simulink model "Top6DOFModel"  (R2018b)
settings: Solver=FixedStepAuto  StartTime=0.0  StopTime=70  FixedStep=0.005  RelTol=1e-3  EnableMultiTasking=on
InitFcn:
  | loadThrusterData
  | loadSensorData
values from neighbouring files (symbols this model uses):
  cameraVec = [1 0 0]    [loadSensorData.m]
  controlRate = 0.025    [loadBusData.m]
  controlType = 1    [loadBusData.m]    (also in loadControlData.m = 2)
  dynamicsRate = 0.005    [loadBusData.m]
  Kd = [x(4) x(5) 0 0 0 x(6)]    [executeSim.m]    (also in loadBusData.m = [500.0000  501.0938 0 0 0 18.4778]; loadControlData.m = [80 80 0 0 0 5] .*[.2 .2  0 0 0 .1]; planarPIDControl.m = [kd(1) 0 0; 0 kd(2) 0; 0 0 kd(3)])
  Ki = [x(7) x(8) 0 0 0 x(9)]    [executeSim.m]    (also in loadBusData.m = [1.0000    1.0313   0 0 0 58.1181]; loadControlData.m = [4  4  0 0 0 1] .*[1   1  0 0 0 .5]; planarPIDControl.m = [ki(1) 0 0; 0 ki(2) 0; 0 0 ki(3)])
  Kp = [x(1) x(2) 0 0 0 x(3)]    [executeSim.m]    (also in loadBusData.m = [500.0000  246.1321 0 0 0 50.1701]; loadControlData.m = [70 70 0 0 0 20].*[.2 .2  0 0 0 .25]; planarPIDControl.m = [kp(1) 0 0; 0 kp(2) 0; 0 0 kp(3)])
  rangeSensorAngBody = [0; 90*dtr; 180*dtr; 270*dtr]    [loadSensorData.m]
  rangeSensorFOV = [0*dtr; 0*dtr; 0*dtr; 0*dtr]    [loadSensorData.m]
  SMGains = x    [executeSim.m]    (also in loadBusData.m = [2.0801    3.0489    8.9333    4.9881    3.0029    9.5293   ; loadControlData.m = [3.5078    3.9888    6.3119    1.8214    4.7749    7.3059   )
  wallBounds = [wallA; wallB; wallC; wallD]    [loadSensorData.m]
undefined symbols (not defined in the file or in its folder): rangeSensorLocBody, targetVec
libraries: simulink x12
settings Model: Creator=Andy  LastModifiedBy=barthal
settings SolverCC: PositivePriorityOrder=on
settings DataIOCC: Decimation=5  SaveFormat=StructureWithTime
settings OptimizationCC: EnhancedBackFolding=on  PassReuseOutputArgsAs=Individual arguments  MaxStackSize=64  OptimizeBlockOrder=speed  DifferentSizesBufferReuse=on  OptimizationCustomize=off
settings DebuggingCC: ParameterTunabilityLossMsg=error
settings HardwareCC: ProdBitPerPointer=32  ProdBitPerSizeT=32  ProdBitPerPtrDiffT=32  ProdLargestAtomicInteger=Long  ProdLargestAtomicFloat=Double  ProdWordSize=32  ProdHWDeviceType=ARM Compatible->ARM Cortex
settings ModelReferenceCC: ModelReferenceNumInstancesAllowed=Single
settings RTWCC: SystemTargetFile=ert.tlc  HardwareBoard=Raspberry Pi  TLCOptions="-aInlineSetEventsForThisBaseRateFcn=TLC_FALSE -aSuppressMultiTaskScheduler=TLC_FALSE  -aRateBasedStepFcn=0"  GenCodeOnly=on  TemplateMakefile=ert_default_tmf  GenerateReport=on  Toolchain=GNU GCC Raspberry Pi  BuildConfiguration=Faster Runs  IncludeHyperlinkInReport=on  LaunchReport=on  TargetLang=C++  GenerateTraceInfo=on  GenerateTraceReport=on  GenerateTraceReportSl=on  GenerateTraceReportSf=on  GenerateTraceReportEml=on
settings CodeAppCC: ForceParamTrailComments=on  IgnoreCustomStorageClasses=off  OperatorAnnotations=on  SimulinkDataObjDesc=on  SFDataObjDesc=on  InsertBlockDesc=on
settings ERTTargetCC: TargetLangStandard=C++03 (ISO)  MatFileLogging=on  MultiInstanceERTCode=on  CodeInterfacePackaging=C++ class  SupportVariableSizeSignals=on  MultiInstanceErrorCode=Warning  RootIOFormat=Structure reference

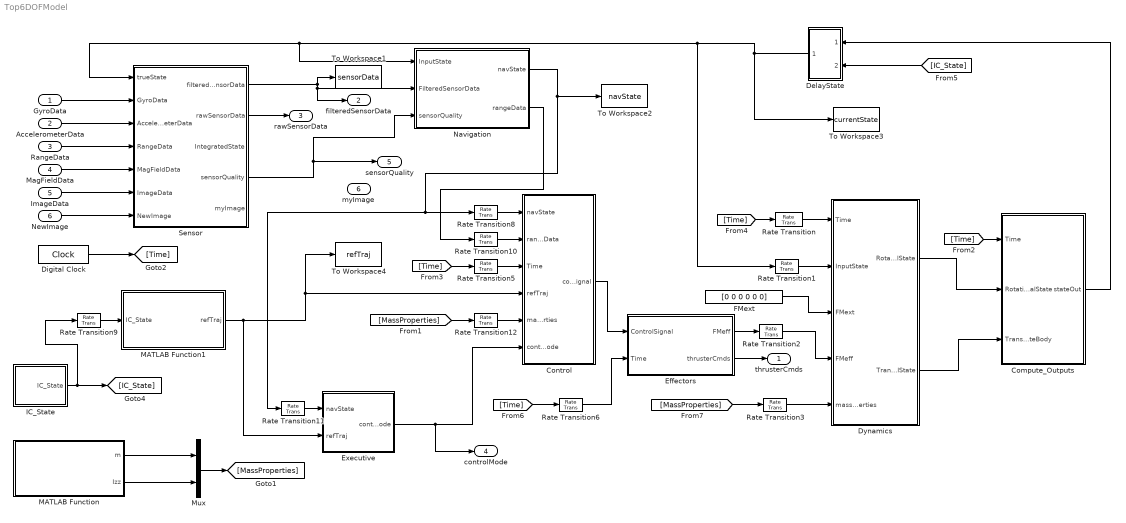
== system Top6DOFModel ==
  GyroData : Inport
  AccelerometerData : Inport  Port=2
  RangeData : Inport  Port=3  OutDataTypeStr=uint8
  MagFieldData : Inport  Port=4
  ImageData : Inport  Port=5  OutDataTypeStr=uint8  PortDimensions=[307200]
  NewImage : Inport  Port=6  OutDataTypeStr=uint8  PortDimensions=[1]
  Compute_Outputs : Subsystem
  Control : Subsystem
  DelayState : Subsystem
  Digital Clock : DigitalClock  SampleTime=0.005
  Dynamics : Subsystem  TreatAsAtomicUnit=on  SystemSampleTime=dynamicsRate
      settings: MinAlgLoopOccurrences=on
  Effectors : Subsystem  TreatAsAtomicUnit=on
  Executive : Subsystem  TreatAsAtomicUnit=on  SystemSampleTime=controlRate
  FMext : Constant  Value=[0 0 0 0 0 0]
  IC_State : Subsystem
  MATLAB Function : MATLAB Function  TreatAsAtomicUnit=on
  MATLAB Function1 : MATLAB Function  TreatAsAtomicUnit=on  SystemSampleTime=controlRate
  Mux : Mux  Inputs=2
  Navigation : Subsystem
  Rate Transition{,1..3} (4 alike) : RateTransition  OutPortSampleTime=dynamicsRate
  Rate Transition{5..6,8..12} (7 alike) : RateTransition  OutPortSampleTime=controlRate
  Sensor : Subsystem
  To Workspace1 : ToWorkspace  VariableName=sensorData  SaveFormat=Timeseries  SampleTime=-1
  To Workspace2 : ToWorkspace  VariableName=navState  SaveFormat=Timeseries  SampleTime=-1
  To Workspace3 : ToWorkspace  VariableName=currentState  SaveFormat=Timeseries  SampleTime=-1
  To Workspace4 : ToWorkspace  VariableName=refTraj  SaveFormat=Timeseries  SampleTime=-1
  thrusterCmds : Outport
  filteredSensorData : Outport  Port=2  OutDataTypeStr=double
  rawSensorData : Outport  Port=3  OutDataTypeStr=double
  controlMode : Outport  Port=4
  sensorQuality : Outport  Port=5
  myImage : Outport  Port=6
  wires:
  Digital Clock/1 -> [Time]
  FMext/1 -> Dynamics/3(FMext)
  Control/1(controlSignal) -> Effectors/1(ControlSignal)
  Dynamics/1(RotationalState) -> Compute_Outputs/2(RotationalState)
  Rate Transition/1 -> Dynamics/1(Time)
  Rate Transition1/1 -> Dynamics/2(InputState)
  Effectors/1(FMeff) -> Rate Transition2/1
  Rate Transition2/1 -> Dynamics/4(FMeff)
  Rate Transition3/1 -> Dynamics/5(massProperties)
  Rate Transition5/1 -> Control/3(Time)
  Rate Transition6/1 -> Effectors/2(Time)
  Dynamics/2(TranslationalState) -> Compute_Outputs/3(TranslationalStateBody)
  IC_State/1(IC_State) -> [IC_State], Rate Transition9/1
  Compute_Outputs/1(stateOut) -> DelayState/1(In4)
  [IC_State] -> DelayState/2(In12)
  DelayState/1(Out4) -> Rate Transition1/1, Navigation/1(InputState), Sensor/1(trueState), To Workspace3/1
  [Time] -> Compute_Outputs/1(Time)
  Rate Transition8/1 -> Control/1(navState)
  MATLAB Function1/1(refTraj) -> To Workspace4/1, Control/4(refTraj), Executive/2(refTraj)
  Effectors/2(thrusterCmds) -> thrusterCmds/1
  GyroData/1 -> Sensor/2(GyroData)
  AccelerometerData/1 -> Sensor/3(AccelerometerData)
  RangeData/1 -> Sensor/4(RangeData)
  Sensor/1(filteredSensorData) -> filteredSensorData/1, Navigation/2(FilteredSensorData), To Workspace1/1
  Executive/1(controlMode) -> Control/6(controlMode), controlMode/1
  Rate Transition11/1 -> Executive/1(navState)
  Rate Transition9/1 -> MATLAB Function1/1(IC_State)
  Rate Transition10/1 -> Control/2(rangeData)
  [Time] -> Rate Transition5/1
  MagFieldData/1 -> Sensor/5(MagFieldData)
  Navigation/1(navState) -> To Workspace2/1, Rate Transition11/1, Rate Transition8/1
  Navigation/2(rangeData) -> Rate Transition10/1
  [Time] -> Rate Transition/1
  [Time] -> Rate Transition6/1
  Sensor/2(rawSensorData) -> rawSensorData/1
  Rate Transition12/1 -> Control/5(massProperties)
  Mux/1 -> [MassProperties]
  [MassProperties] -> Rate Transition12/1
  [MassProperties] -> Rate Transition3/1
  MATLAB Function/1(m) -> Mux/1
  MATLAB Function/2(Izz) -> Mux/2
  Sensor/4(sensorQuality) -> sensorQuality/1, Navigation/3(sensorQuality)
  ImageData/1 -> Sensor/6(ImageData)
  NewImage/1 -> Sensor/7(NewImage)

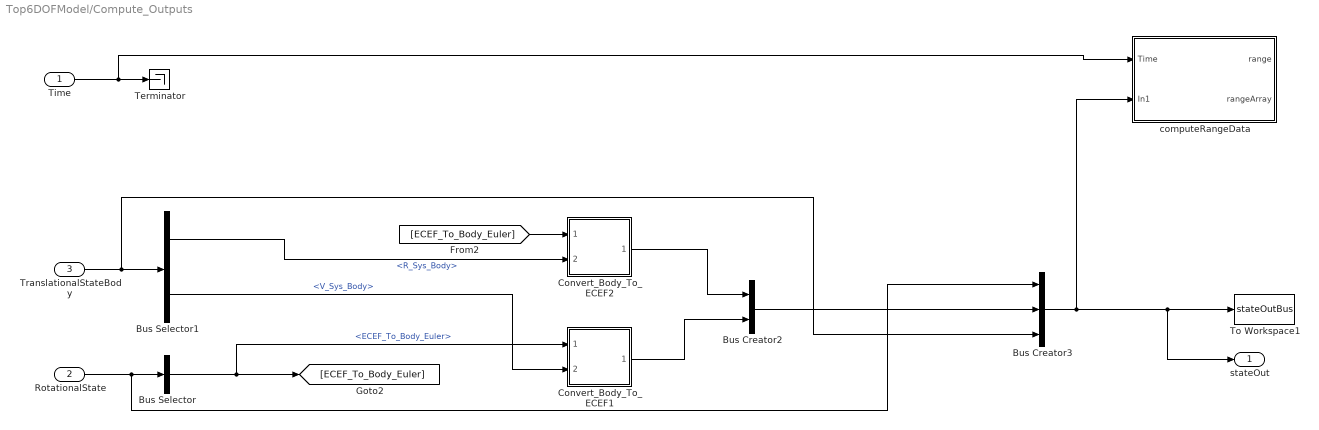
== system Top6DOFModel/Compute_Outputs ==
  Time : Inport
  RotationalState : Inport  Port=2
  TranslationalStateBody : Inport  Port=3
  Bus Creator2 : BusCreator  Inputs=2  OutDataTypeStr=Bus: TranStateECEFBus
      settings: InheritFromInputs=off
  Bus Creator3 : BusCreator  Inputs=3  OutDataTypeStr=Bus: FullStateBus
      settings: InheritFromInputs=off
  Bus Selector : BusSelector  OutputSignals=ECEF_To_Body_Euler
  Bus Selector1 : BusSelector  OutputSignals=R_Sys_Body,V_Sys_Body
  Convert_Body_To_ECEF1 : Subsystem
  Convert_Body_To_ECEF2 : Subsystem
  Terminator : Terminator
  To Workspace1 : ToWorkspace  VariableName=stateOutBus  SaveFormat=Timeseries  SampleTime=-1
  computeRangeData : Subsystem
  stateOut : Outport
  wires:
  RotationalState/1 -> Bus Creator3/1, Bus Selector/1
  Bus Selector/1 -> Convert_Body_To_ECEF1/1(ECEF_To_Body_Euler), [ECEF_To_Body_Euler]  "<ECEF_To_Body_Euler>"
  Convert_Body_To_ECEF2/1(Vec_ECEF) -> Bus Creator2/1
  Convert_Body_To_ECEF1/1(Vec_ECEF) -> Bus Creator2/2
  [ECEF_To_Body_Euler] -> Convert_Body_To_ECEF2/1(ECEF_To_Body_Euler)
  TranslationalStateBody/1 -> Bus Creator3/3, Bus Selector1/1
  Bus Selector1/1 -> Convert_Body_To_ECEF2/2(Vec_Body)  "<R_Sys_Body>"
  Bus Selector1/2 -> Convert_Body_To_ECEF1/2(Vec_Body)  "<V_Sys_Body>"
  Bus Creator2/1 -> Bus Creator3/2
  Bus Creator3/1 -> stateOut/1, To Workspace1/1, computeRangeData/2(In1)
  Time/1 -> computeRangeData/1(Time), Terminator/1

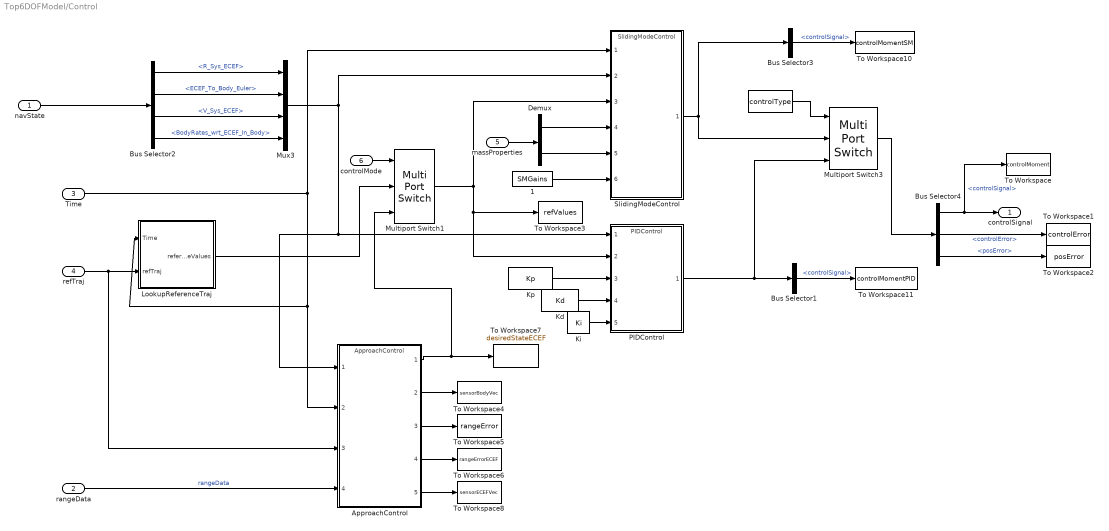
== system Top6DOFModel/Control ==
  navState : Inport
  rangeData : Inport  Port=2
  Time : Inport  Port=3
  refTraj : Inport  Port=4
  massProperties : Inport  Port=5
  controlMode : Inport  Port=6
  " " : Constant  Value=controlType
  " 1" : Constant  Value=SMGains
  ApproachControl : ModelReference  ModelNameDialog=ApproachControl  SimulationMode=Normal  ModelReferenceVersion=1.58
  Bus Selector1 : BusSelector  OutputSignals=controlSignal
  Bus Selector2 : BusSelector  OutputSignals=TranState_ECEF.R_Sys_ECEF,RotState_Body_ECEF.ECEF_To_Body_Euler,TranState_ECEF.V_Sys_ECEF,RotState_Body_ECEF.BodyRates_wrt_ECEF_In_Body
  Bus Selector3 : BusSelector  OutputSignals=controlSignal
  Bus Selector4 : BusSelector  OutputSignals=controlSignal,controlError,posError
  Demux : Demux  Outputs=2
  Kd : Constant  Value=Kd
  Ki : Constant  Value=Ki
  Kp : Constant  Value=Kp
  LookupReferenceTraj : Subsystem
  Multiport Switch1 : MultiPortSwitch  Inputs=2
  Multiport Switch3 : MultiPortSwitch  Inputs=2
  Mux3 : Mux
  PIDControl : ModelReference  ModelNameDialog=PIDControl  SimulationMode=Normal  ModelReferenceVersion=1.353
  SlidingModeControl : ModelReference  ModelNameDialog=SlidingModeControl  SimulationMode=Normal  ModelReferenceVersion=1.17
  To Workspace : ToWorkspace  VariableName=controlMoment  SaveFormat=Timeseries  SampleTime=-1
  To Workspace1 : ToWorkspace  VariableName=controlError  SaveFormat=Timeseries  SampleTime=-1
  To Workspace10 : ToWorkspace  VariableName=controlMomentSM  SaveFormat=Timeseries  SampleTime=-1
  To Workspace11 : ToWorkspace  VariableName=controlMomentPID  SaveFormat=Timeseries  SampleTime=-1
  To Workspace2 : ToWorkspace  VariableName=posError  SaveFormat=Timeseries  SampleTime=-1
  To Workspace3 : ToWorkspace  VariableName=refValues  SaveFormat=Timeseries  SampleTime=-1
  To Workspace4 : ToWorkspace  VariableName=sensorBodyVec  SaveFormat=Timeseries  SampleTime=-1
  To Workspace5 : ToWorkspace  VariableName=rangeError  SaveFormat=Timeseries  SampleTime=-1
  To Workspace6 : ToWorkspace  VariableName=rangeErrorECEF  SaveFormat=Timeseries  SampleTime=-1
  To Workspace7 : ToWorkspace  VariableName=desiredStateECEF  SaveFormat=Timeseries  SampleTime=-1
  To Workspace8 : ToWorkspace  VariableName=sensorECEFVec  SaveFormat=Timeseries  SampleTime=-1
  controlSignal : Outport
  wires:
  refTraj/1 -> LookupReferenceTraj/2(refTraj), ApproachControl/3
  Mux3/1 -> SlidingModeControl/2, PIDControl/1, ApproachControl/1
  navState/1 -> Bus Selector2/1
  Bus Selector2/1 -> Mux3/1  "<R_Sys_ECEF>"
  Bus Selector2/2 -> Mux3/2  "<ECEF_To_Body_Euler>"
  Bus Selector2/3 -> Mux3/3  "<V_Sys_ECEF>"
  Bus Selector2/4 -> Mux3/4  "<BodyRates_wrt_ECEF_In_Body>"
  rangeData/1 -> ApproachControl/4  "rangeData"
  Time/1 -> ApproachControl/2, LookupReferenceTraj/1(Time), SlidingModeControl/1
  Kp/1 -> PIDControl/3
  Kd/1 -> PIDControl/4
  Ki/1 -> PIDControl/5
  Demux/2 -> SlidingModeControl/5
  SlidingModeControl/1 -> Bus Selector3/1, Multiport Switch3/2
  " "/1 -> Multiport Switch3/1
  PIDControl/1 -> Bus Selector1/1, Multiport Switch3/3
  Multiport Switch3/1 -> Bus Selector4/1
  Bus Selector4/1 -> To Workspace/1, controlSignal/1  "<controlSignal>"
  Bus Selector4/2 -> To Workspace1/1  "<controlError>"
  Bus Selector4/3 -> To Workspace2/1  "<posError>"
  Bus Selector1/1 -> To Workspace11/1  "<controlSignal>"
  Bus Selector3/1 -> To Workspace10/1  "<controlSignal>"
  " 1"/1 -> SlidingModeControl/6
  controlMode/1 -> Multiport Switch1/1
  Multiport Switch1/1 -> To Workspace3/1, PIDControl/2, SlidingModeControl/3
  LookupReferenceTraj/1(referenceValues) -> Multiport Switch1/2
  ApproachControl/1 -> Multiport Switch1/3, To Workspace7/1
  ApproachControl/2 -> To Workspace4/1
  ApproachControl/3 -> To Workspace5/1
  ApproachControl/4 -> To Workspace6/1
  ApproachControl/5 -> To Workspace8/1
  Demux/1 -> SlidingModeControl/4
  massProperties/1 -> Demux/1

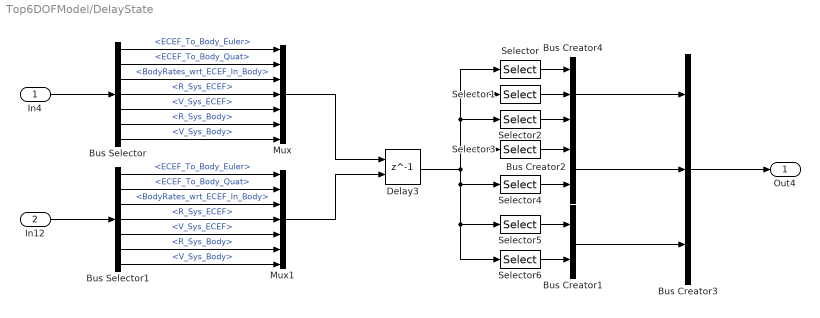
== system Top6DOFModel/DelayState ==
  In4 : Inport
  In12 : Inport  Port=2
  Bus Creator1 : BusCreator  Inputs=2  OutDataTypeStr=Bus: TranStateBodyBus
      settings: InheritFromInputs=off
  Bus Creator2 : BusCreator  Inputs=2  OutDataTypeStr=Bus: TranStateECEFBus
      settings: InheritFromInputs=off
  Bus Creator3 : BusCreator  Inputs=3  OutDataTypeStr=Bus: FullStateBus
      settings: InheritFromInputs=off
  Bus Creator4 : BusCreator  Inputs=3  OutDataTypeStr=Bus: RotStateBodyECEFBus
      settings: InheritFromInputs=off
  Bus Selector : BusSelector  OutputSignals=RotState_Body_ECEF.ECEF_To_Body_Euler,RotState_Body_ECEF.ECEF_To_Body_Quat,RotState_Body_ECEF.BodyRates_wrt_ECEF_In_Body,TranState_ECEF.R_Sys_ECEF,TranState_ECEF.V_Sys_ECEF,TranState_Body.R_Sys_Body,TranState_Body.V_Sys_Body
  Bus Selector1 : BusSelector  OutputSignals=RotState_Body_ECEF.ECEF_To_Body_Euler,RotState_Body_ECEF.ECEF_To_Body_Quat,RotState_Body_ECEF.BodyRates_wrt_ECEF_In_Body,TranState_ECEF.R_Sys_ECEF,TranState_ECEF.V_Sys_ECEF,TranState_Body.R_Sys_Body,TranState_Body.V_Sys_Body
  Delay3 : Delay  DelayLength=1  InitialConditionSource=Input port
      settings: InputPortMap=u0,p4
  Mux : Mux  Inputs=7
  Mux1 : Mux  Inputs=7
  Selector : Selector  InputPortWidth=22  IndexOptions=Index vector (dialog)  Indices=[1:3]  OutputSizes=1
  Selector1 : Selector  InputPortWidth=22  IndexOptions=Index vector (dialog)  Indices=[4:7]  OutputSizes=1
  Selector2 : Selector  InputPortWidth=22  IndexOptions=Index vector (dialog)  Indices=[8:10]  OutputSizes=1
  Selector3 : Selector  InputPortWidth=22  IndexOptions=Index vector (dialog)  Indices=[11:13]  OutputSizes=1
  Selector4 : Selector  InputPortWidth=22  IndexOptions=Index vector (dialog)  Indices=[14:16]  OutputSizes=1
  Selector5 : Selector  InputPortWidth=22  IndexOptions=Index vector (dialog)  Indices=[17:19]  OutputSizes=1
  Selector6 : Selector  InputPortWidth=22  IndexOptions=Index vector (dialog)  Indices=[20:22]  OutputSizes=1
  Out4 : Outport
  wires:
  Bus Creator3/1 -> Out4/1
  Bus Creator1/1 -> Bus Creator3/3
  Bus Creator2/1 -> Bus Creator3/2
  Bus Creator4/1 -> Bus Creator3/1
  In4/1 -> Bus Selector/1
  Bus Selector/1 -> Mux/1  "<ECEF_To_Body_Euler>"
  Bus Selector/2 -> Mux/2  "<ECEF_To_Body_Quat>"
  Bus Selector/3 -> Mux/3  "<BodyRates_wrt_ECEF_In_Body>"
  Bus Selector/4 -> Mux/4  "<R_Sys_ECEF>"
  Bus Selector/5 -> Mux/5  "<V_Sys_ECEF>"
  Bus Selector/6 -> Mux/6  "<R_Sys_Body>"
  Bus Selector/7 -> Mux/7  "<V_Sys_Body>"
  Bus Selector1/4 -> Mux1/4  "<R_Sys_ECEF>"
  Bus Selector1/2 -> Mux1/2  "<ECEF_To_Body_Quat>"
  Bus Selector1/1 -> Mux1/1  "<ECEF_To_Body_Euler>"
  In12/1 -> Bus Selector1/1
  Bus Selector1/6 -> Mux1/6  "<R_Sys_Body>"
  Bus Selector1/5 -> Mux1/5  "<V_Sys_ECEF>"
  Bus Selector1/7 -> Mux1/7  "<V_Sys_Body>"
  Bus Selector1/3 -> Mux1/3  "<BodyRates_wrt_ECEF_In_Body>"
  Mux/1 -> Delay3/1
  Mux1/1 -> Delay3/2
  Selector/1 -> Bus Creator4/1
  Selector1/1 -> Bus Creator4/2
  Selector2/1 -> Bus Creator4/3
  Selector3/1 -> Bus Creator2/1
  Selector4/1 -> Bus Creator2/2
  Selector5/1 -> Bus Creator1/1
  Selector6/1 -> Bus Creator1/2
  Delay3/1 -> Selector/1, Selector1/1, Selector2/1, Selector3/1, Selector4/1, Selector5/1, Selector6/1

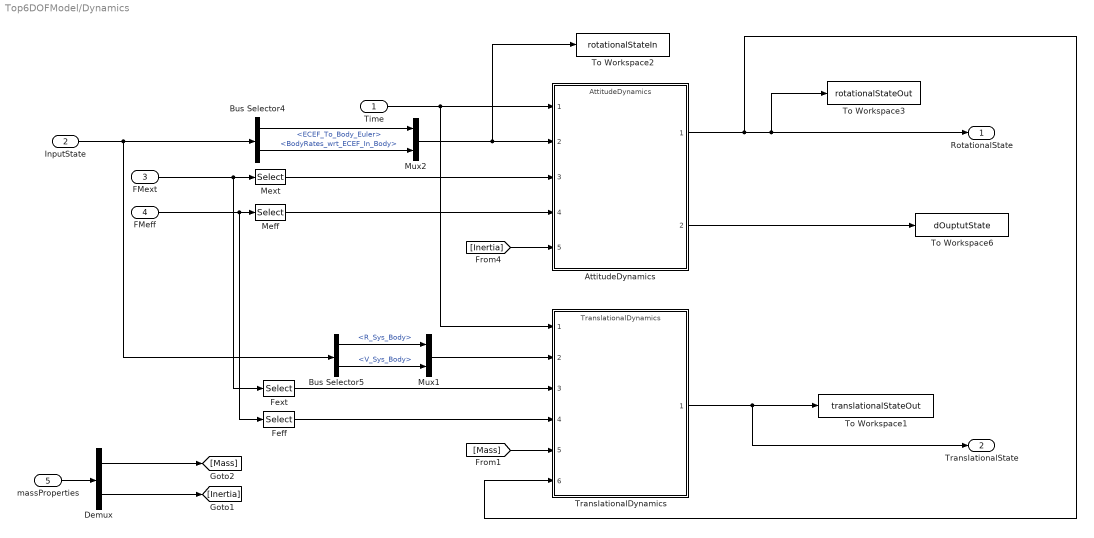
== system Top6DOFModel/Dynamics ==
  Time : Inport
  InputState : Inport  Port=2
  FMext : Inport  Port=3
  FMeff : Inport  Port=4
  massProperties : Inport  Port=5
  AttitudeDynamics : ModelReference  ModelNameDialog=AttitudeDynamics  SimulationMode=Normal  ModelReferenceVersion=1.377
  Bus Selector4 : BusSelector  OutputSignals=RotState_Body_ECEF.ECEF_To_Body_Euler,RotState_Body_ECEF.BodyRates_wrt_ECEF_In_Body
  Bus Selector5 : BusSelector  OutputSignals=TranState_Body.R_Sys_Body,TranState_Body.V_Sys_Body
  Demux : Demux  Outputs=2
  Feff : Selector  InputPortWidth=6  IndexOptions=Index vector (dialog)  Indices=[1:3]  OutputSizes=1
  Fext : Selector  InputPortWidth=6  IndexOptions=Index vector (dialog)  Indices=[1:3]  OutputSizes=1
  Meff : Selector  InputPortWidth=6  IndexOptions=Index vector (dialog)  Indices=[4:6]  OutputSizes=1
  Mext : Selector  InputPortWidth=6  IndexOptions=Index vector (dialog)  Indices=[4:6]  OutputSizes=1
  Mux1 : Mux  Inputs=2
  Mux2 : Mux  Inputs=2
  To Workspace1 : ToWorkspace  VariableName=translationalStateOut  SaveFormat=Timeseries  SampleTime=-1
  To Workspace2 : ToWorkspace  VariableName=rotationalStateIn  SaveFormat=Timeseries  SampleTime=-1
  To Workspace3 : ToWorkspace  VariableName=rotationalStateOut  SaveFormat=Timeseries  SampleTime=-1
  To Workspace6 : ToWorkspace  VariableName=dOuptutState  SaveFormat=Timeseries  SampleTime=-1
  TranslationalDynamics : ModelReference  ModelNameDialog=TranslationalDynamics  SimulationMode=Normal  ModelReferenceVersion=1.363
  RotationalState : Outport
  TranslationalState : Outport  Port=2
  wires:
  Time/1 -> AttitudeDynamics/1, TranslationalDynamics/1
  FMext/1 -> Mext/1, Fext/1
  Mext/1 -> AttitudeDynamics/3
  Fext/1 -> TranslationalDynamics/3
  FMeff/1 -> Feff/1, Meff/1
  Feff/1 -> TranslationalDynamics/4
  Meff/1 -> AttitudeDynamics/4
  AttitudeDynamics/2 -> To Workspace6/1
  AttitudeDynamics/1 -> RotationalState/1, To Workspace3/1, TranslationalDynamics/6
  TranslationalDynamics/1 -> TranslationalState/1, To Workspace1/1
  InputState/1 -> Bus Selector5/1, Bus Selector4/1
  Bus Selector4/1 -> Mux2/1  "<ECEF_To_Body_Euler>"
  Bus Selector4/2 -> Mux2/2  "<BodyRates_wrt_ECEF_In_Body>"
  Mux1/1 -> TranslationalDynamics/2
  Mux2/1 -> To Workspace2/1, AttitudeDynamics/2
  Bus Selector5/1 -> Mux1/1  "<R_Sys_Body>"
  Bus Selector5/2 -> Mux1/2  "<V_Sys_Body>"
  massProperties/1 -> Demux/1
  [Inertia] -> AttitudeDynamics/5
  [Mass] -> TranslationalDynamics/5
  Demux/1 -> [Mass]
  Demux/2 -> [Inertia]

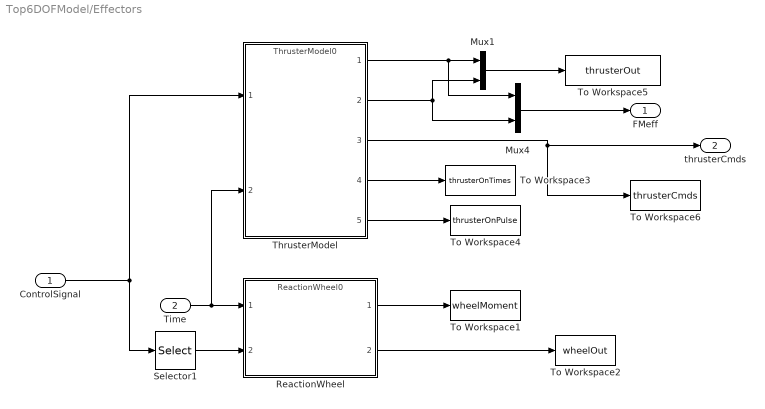
== system Top6DOFModel/Effectors ==
  ControlSignal : Inport
  Time : Inport  Port=2
  Mux1 : Mux  Inputs=2
  Mux4 : Mux  Inputs=2
  ReactionWheel : ModelReference  ModelNameDialog=ReactionWheel0  SimulationMode=Normal  ModelReferenceVersion=1.304
  Selector1 : Selector  InputPortWidth=6  IndexOptions=Index vector (dialog)  Indices=[6]  OutputSizes=1
  ThrusterModel : ModelReference  ModelNameDialog=ThrusterModel0  SimulationMode=Normal  ModelReferenceVersion=1.328
  To Workspace1 : ToWorkspace  VariableName=wheelMoment  SaveFormat=Timeseries  SampleTime=-1
  To Workspace2 : ToWorkspace  VariableName=wheelOut  SaveFormat=Timeseries  SampleTime=-1
  To Workspace3 : ToWorkspace  VariableName=thrusterOnTimes  SaveFormat=Timeseries  SampleTime=-1
  To Workspace4 : ToWorkspace  VariableName=thrusterOnPulse  SaveFormat=Timeseries  SampleTime=-1
  To Workspace5 : ToWorkspace  VariableName=thrusterOut  SaveFormat=Timeseries  SampleTime=-1
  To Workspace6 : ToWorkspace  VariableName=thrusterCmds  SaveFormat=Timeseries  SampleTime=-1
  FMeff : Outport
  thrusterCmds : Outport  Port=2
  wires:
  Selector1/1 -> ReactionWheel/2
  ControlSignal/1 -> ThrusterModel/1, Selector1/1
  Time/1 -> ThrusterModel/2, ReactionWheel/1
  Mux4/1 -> FMeff/1
  ThrusterModel/3 -> To Workspace6/1, thrusterCmds/1
  ReactionWheel/1 -> To Workspace1/1
  ReactionWheel/2 -> To Workspace2/1
  ThrusterModel/2 -> Mux4/2, Mux1/2
  ThrusterModel/1 -> Mux4/1, Mux1/1
  Mux1/1 -> To Workspace5/1
  ThrusterModel/4 -> To Workspace3/1
  ThrusterModel/5 -> To Workspace4/1

== system Top6DOFModel/Executive ==
  navState : Inport
  refTraj : Inport  Port=2
  Constant : Constant
  Delay : Delay  DelayLength=1  InitialConditionSource=Input port  InitialCondition=0
      settings: InputPortMap=u0,p4
  MATLAB Function : MATLAB Function  TreatAsAtomicUnit=on
  To Workspace2 : ToWorkspace  VariableName=controlMode  SaveFormat=Timeseries  SampleTime=-1
  controlMode : Outport
  wires:
  Delay/1 -> MATLAB Function/3(inControlMode)
  refTraj/1 -> MATLAB Function/2(refTraj)
  navState/1 -> MATLAB Function/1(navState)
  MATLAB Function/1(outControlMode) -> To Workspace2/1, controlMode/1, Delay/1
  Constant/1 -> Delay/2

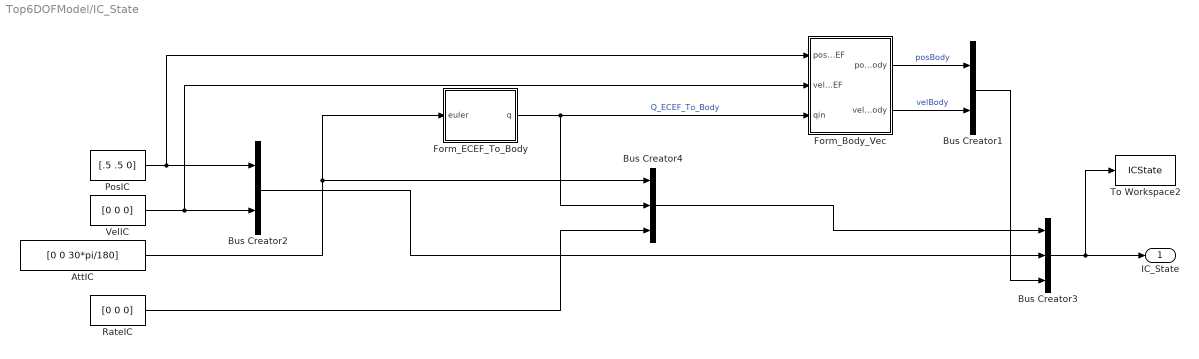
== system Top6DOFModel/IC_State ==
  AttIC : Constant  Value=[0 0 30*pi/180]
  Bus Creator1 : BusCreator  Inputs=2  OutDataTypeStr=Bus: TranStateBodyBus
      settings: InheritFromInputs=off
  Bus Creator2 : BusCreator  Inputs=2  OutDataTypeStr=Bus: TranStateECEFBus
      settings: InheritFromInputs=off
  Bus Creator3 : BusCreator  Inputs=3  OutDataTypeStr=Bus: FullStateBus
      settings: InheritFromInputs=off
  Bus Creator4 : BusCreator  Inputs=3  OutDataTypeStr=Bus: RotStateBodyECEFBus
      settings: InheritFromInputs=off
  Form_Body_Vec : MATLAB Function  TreatAsAtomicUnit=on
  Form_ECEF_To_Body : MATLAB Function  TreatAsAtomicUnit=on
  PosIC : Constant  Value=[.5 .5 0]
  RateIC : Constant  Value=[0 0 0]
  To Workspace2 : ToWorkspace  VariableName=ICState  SaveFormat=Timeseries  SampleTime=-1
  VelIC : Constant  Value=[0 0 0]
  IC_State : Outport
  wires:
  RateIC/1 -> Bus Creator4/3
  PosIC/1 -> Form_Body_Vec/1(posECEF), Bus Creator2/1
  VelIC/1 -> Bus Creator2/2, Form_Body_Vec/2(velECEF)
  Form_ECEF_To_Body/1(q) -> Form_Body_Vec/3(qin), Bus Creator4/2  "Q_ECEF_To_Body"
  Form_Body_Vec/1(posBody) -> Bus Creator1/1  "posBody"
  Form_Body_Vec/2(velBody) -> Bus Creator1/2  "velBody"
  Bus Creator2/1 -> Bus Creator3/2
  Bus Creator1/1 -> Bus Creator3/3
  Bus Creator4/1 -> Bus Creator3/1
  Bus Creator3/1 -> To Workspace2/1, IC_State/1
  AttIC/1 -> Bus Creator4/1, Form_ECEF_To_Body/1(euler)

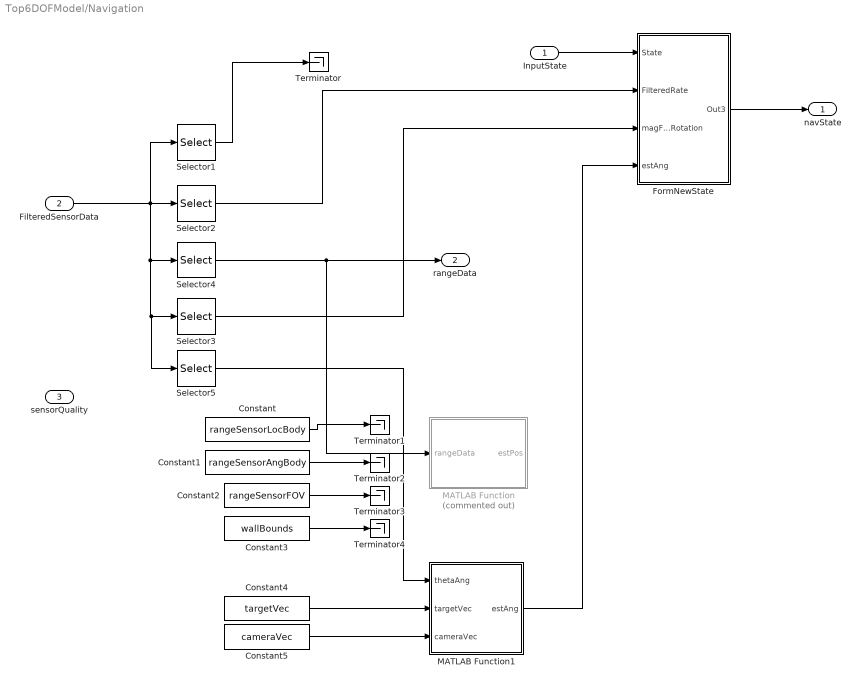
== system Top6DOFModel/Navigation ==
  InputState : Inport
  FilteredSensorData : Inport  Port=2
  sensorQuality : Inport  Port=3
  Constant : Constant  Value=rangeSensorLocBody
  Constant1 : Constant  Value=rangeSensorAngBody
  Constant2 : Constant  Value=rangeSensorFOV
  Constant3 : Constant  Value=wallBounds
  Constant4 : Constant  Value=targetVec
  Constant5 : Constant  Value=cameraVec
  FormNewState : Subsystem
  MATLAB Function : MATLAB Function  Commented=on  TreatAsAtomicUnit=on
  MATLAB Function1 : MATLAB Function  TreatAsAtomicUnit=on
  Selector1 : Selector  InputPortWidth=14  IndexOptions=Index vector (dialog)  Indices=[1:3]  OutputSizes=1
  Selector2 : Selector  InputPortWidth=14  IndexOptions=Index vector (dialog)  Indices=[4:6]  OutputSizes=1
  Selector3 : Selector  InputPortWidth=14  IndexOptions=Index vector (dialog)  Indices=[11:13]  OutputSizes=1
  Selector4 : Selector  InputPortWidth=14  IndexOptions=Index vector (dialog)  Indices=[7:10]  OutputSizes=1
  Selector5 : Selector  InputPortWidth=14  IndexOptions=Index vector (dialog)  Indices=[14]  OutputSizes=1
  Terminator{,1..4} (5 alike) : Terminator
  navState : Outport
  rangeData : Outport  Port=2
  wires:
  FilteredSensorData/1 -> Selector4/1, Selector5/1, Selector3/1, Selector2/1, Selector1/1
  Selector2/1 -> FormNewState/2(FilteredRate)
  Selector3/1 -> FormNewState/3(magFieldRotation)
  InputState/1 -> FormNewState/1(State)
  FormNewState/1(Out3) -> navState/1
  Selector4/1 -> MATLAB Function/1(rangeData), rangeData/1
  Constant3/1 -> Terminator4/1
  Constant2/1 -> Terminator3/1
  Constant1/1 -> Terminator2/1
  Constant/1 -> Terminator1/1
  Selector1/1 -> Terminator/1
  Selector5/1 -> MATLAB Function1/1(thetaAng)
  Constant4/1 -> MATLAB Function1/2(targetVec)
  MATLAB Function1/1(estAng) -> FormNewState/4(estAng)
  Constant5/1 -> MATLAB Function1/3(cameraVec)

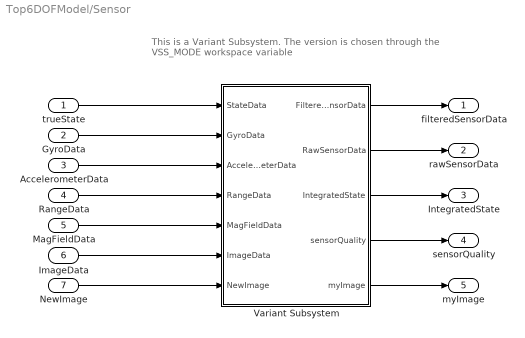
== system Top6DOFModel/Sensor ==
  note: This is a Variant Subsystem.
      | The version is chosen through the VSS_MODE workspace variable
  trueState : Inport  OutDataTypeStr=double
  GyroData : Inport  Port=2  OutDataTypeStr=double
  AccelerometerData : Inport  Port=3  OutDataTypeStr=double
  RangeData : Inport  Port=4  OutDataTypeStr=uint8
  MagFieldData : Inport  Port=5  OutDataTypeStr=double
  ImageData : Inport  Port=6
  NewImage : Inport  Port=7  OutDataTypeStr=uint8
  Variant Subsystem : Subsystem  Variant=on
  filteredSensorData : Outport  OutDataTypeStr=double
  rawSensorData : Outport  Port=2  OutDataTypeStr=double
  IntegratedState : Outport  Port=3  OutDataTypeStr=double
  sensorQuality : Outport  Port=4
  myImage : Outport  Port=5  OutDataTypeStr=uint8
  wires:
  trueState/1 -> Variant Subsystem/1(StateData)
  GyroData/1 -> Variant Subsystem/2(GyroData)
  AccelerometerData/1 -> Variant Subsystem/3(AccelerometerData)
  RangeData/1 -> Variant Subsystem/4(RangeData)
  Variant Subsystem/1(FilteredSensorData) -> filteredSensorData/1
  MagFieldData/1 -> Variant Subsystem/5(MagFieldData)
  Variant Subsystem/2(RawSensorData) -> rawSensorData/1
  Variant Subsystem/3(IntegratedState) -> IntegratedState/1
  Variant Subsystem/4(sensorQuality) -> sensorQuality/1
  ImageData/1 -> Variant Subsystem/6(ImageData)
  Variant Subsystem/5(myImage) -> myImage/1
  NewImage/1 -> Variant Subsystem/7(NewImage)

== system Top6DOFModel/Compute_Outputs/Convert_Body_To_ECEF1 ==
  ECEF_To_Body_Euler : Inport
  Vec_Body : Inport  Port=2  PortDimensions=3
  Form_ECEF_To_Body : MATLAB Function  TreatAsAtomicUnit=on
  Math Function : Math  Operator=transpose  SaturateOnIntegerOverflow=on
  Product : Product  Multiplication=Matrix(*)
  Terminator : Terminator
  Vec_ECEF : Outport  PortDimensions=3
  wires:
  Form_ECEF_To_Body/1(m) -> Math Function/1  "M_ECEF_To_Body"
  Vec_Body/1 -> Product/2
  Product/1 -> Vec_ECEF/1
  ECEF_To_Body_Euler/1 -> Form_ECEF_To_Body/1(euler)
  Form_ECEF_To_Body/2(q) -> Terminator/1  "q_ECEF_To_Body"
  Math Function/1 -> Product/1

== system Top6DOFModel/Compute_Outputs/Convert_Body_To_ECEF2 ==
  ECEF_To_Body_Euler : Inport
  Vec_Body : Inport  Port=2  PortDimensions=3
  Form_ECEF_To_Body : MATLAB Function  TreatAsAtomicUnit=on
  Math Function : Math  Operator=transpose  SaturateOnIntegerOverflow=on
  Product : Product  Multiplication=Matrix(*)
  Terminator : Terminator
  Vec_ECEF : Outport  PortDimensions=3
  wires:
  Form_ECEF_To_Body/1(m) -> Math Function/1  "M_ECEF_To_Body"
  Vec_Body/1 -> Product/2
  Product/1 -> Vec_ECEF/1
  ECEF_To_Body_Euler/1 -> Form_ECEF_To_Body/1(euler)
  Form_ECEF_To_Body/2(q) -> Terminator/1  "q_ECEF_To_Body"
  Math Function/1 -> Product/1

== system Top6DOFModel/Compute_Outputs/computeRangeData ==
  Time : Inport
  In1 : Inport  Port=2
  Constant : Constant  Value=rangeSensorLocBody
  Constant1 : Constant  Value=rangeSensorAngBody
  Constant2 : Constant  Value=rangeSensorFOV
  Constant3 : Constant  Value=wallBounds
  MATLAB Function1 : MATLAB Function  TreatAsAtomicUnit=on
  range : Outport
  rangeArray : Outport  Port=2
  wires:
  In1/1 -> MATLAB Function1/2(state)
  Constant/1 -> MATLAB Function1/3(rangeSensorLocBody)
  Constant1/1 -> MATLAB Function1/4(rangeSensorAngBody)
  Constant2/1 -> MATLAB Function1/5(rangeSensorFOV)
  MATLAB Function1/1(range) -> range/1
  Constant3/1 -> MATLAB Function1/6(wallBounds)
  MATLAB Function1/2(rangeArray) -> rangeArray/1
  Time/1 -> MATLAB Function1/1(t)

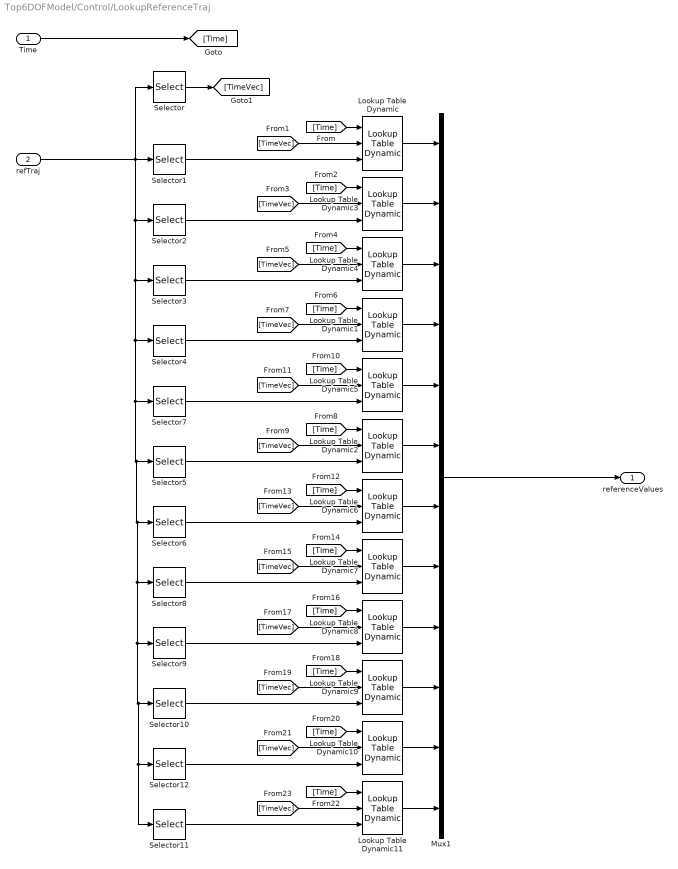
== system Top6DOFModel/Control/LookupReferenceTraj ==
  Time : Inport
  refTraj : Inport  Port=2
  Lookup Table Dynamic{,1..11} (12 alike) : simulink/Lookup Tables/Lookup Table Dynamic  LookUpMeth=Interpolation-Use End Values  OutDataType=fixdt('double')  OutScaling=[]  OutputDataTypeScalingMode=Specify via dialog  OutDataTypeStr=double  DoSatur=off
      settings: SourceProductName=Simulink
  Mux1 : Mux  Inputs=12
  Selector : Selector  NumberOfDimensions=2  InputPortWidth=3  IndexOptions=Select all,Index vector (dialog)  Indices=1,1  OutputSizes=1,1
  Selector1 : Selector  NumberOfDimensions=2  InputPortWidth=3  IndexOptions=Select all,Index vector (dialog)  Indices=1,2  OutputSizes=1,1
  Selector10 : Selector  NumberOfDimensions=2  InputPortWidth=3  IndexOptions=Select all,Index vector (dialog)  Indices=1,11  OutputSizes=1,1
  Selector11 : Selector  NumberOfDimensions=2  InputPortWidth=3  IndexOptions=Select all,Index vector (dialog)  Indices=1,13  OutputSizes=1,1
  Selector12 : Selector  NumberOfDimensions=2  InputPortWidth=3  IndexOptions=Select all,Index vector (dialog)  Indices=1,12  OutputSizes=1,1
  Selector2 : Selector  NumberOfDimensions=2  InputPortWidth=3  IndexOptions=Select all,Index vector (dialog)  Indices=1,3  OutputSizes=1,1
  Selector3 : Selector  NumberOfDimensions=2  InputPortWidth=3  IndexOptions=Select all,Index vector (dialog)  Indices=1,4  OutputSizes=1,1
  Selector4 : Selector  NumberOfDimensions=2  InputPortWidth=3  IndexOptions=Select all,Index vector (dialog)  Indices=1,5  OutputSizes=1,1
  Selector5 : Selector  NumberOfDimensions=2  InputPortWidth=3  IndexOptions=Select all,Index vector (dialog)  Indices=1,7  OutputSizes=1,1
  Selector6 : Selector  NumberOfDimensions=2  InputPortWidth=3  IndexOptions=Select all,Index vector (dialog)  Indices=1,8  OutputSizes=1,1
  Selector7 : Selector  NumberOfDimensions=2  InputPortWidth=3  IndexOptions=Select all,Index vector (dialog)  Indices=1,6  OutputSizes=1,1
  Selector8 : Selector  NumberOfDimensions=2  InputPortWidth=3  IndexOptions=Select all,Index vector (dialog)  Indices=1,9  OutputSizes=1,1
  Selector9 : Selector  NumberOfDimensions=2  InputPortWidth=3  IndexOptions=Select all,Index vector (dialog)  Indices=1,10  OutputSizes=1,1
  referenceValues : Outport
  wires:
  Lookup Table Dynamic2/1 -> Mux1/6
  Lookup Table Dynamic5/1 -> Mux1/5
  Lookup Table Dynamic1/1 -> Mux1/4
  Lookup Table Dynamic/1 -> Mux1/1
  Lookup Table Dynamic3/1 -> Mux1/2
  Lookup Table Dynamic4/1 -> Mux1/3
  Selector7/1 -> Lookup Table Dynamic5/3
  Selector5/1 -> Lookup Table Dynamic2/3
  [TimeVec] -> Lookup Table Dynamic2/2
  [Time] -> Lookup Table Dynamic4/1
  Selector3/1 -> Lookup Table Dynamic4/3
  [Time] -> Lookup Table Dynamic3/1
  Selector2/1 -> Lookup Table Dynamic3/3
  [TimeVec] -> Lookup Table Dynamic4/2
  [Time] -> Lookup Table Dynamic/1
  Selector1/1 -> Lookup Table Dynamic/3
  Mux1/1 -> referenceValues/1
  [TimeVec] -> Lookup Table Dynamic5/2
  Selector/1 -> [TimeVec]
  refTraj/1 -> Selector1/1, Selector/1, Selector2/1, Selector3/1, Selector4/1, Selector7/1, Selector11/1, Selector12/1, Selector10/1, Selector9/1, Selector8/1, Selector6/1, Selector5/1
  [Time] -> Lookup Table Dynamic5/1
  [TimeVec] -> Lookup Table Dynamic3/2
  [Time] -> Lookup Table Dynamic2/1
  [Time] -> Lookup Table Dynamic1/1
  Time/1 -> [Time]
  [TimeVec] -> Lookup Table Dynamic/2
  [TimeVec] -> Lookup Table Dynamic1/2
  Selector4/1 -> Lookup Table Dynamic1/3
  [TimeVec] -> Lookup Table Dynamic6/2
  [Time] -> Lookup Table Dynamic6/1
  Selector6/1 -> Lookup Table Dynamic6/3
  [TimeVec] -> Lookup Table Dynamic7/2
  [Time] -> Lookup Table Dynamic7/1
  Selector8/1 -> Lookup Table Dynamic7/3
  Selector10/1 -> Lookup Table Dynamic9/3
  [Time] -> Lookup Table Dynamic9/1
  [TimeVec] -> Lookup Table Dynamic9/2
  [TimeVec] -> Lookup Table Dynamic8/2
  [Time] -> Lookup Table Dynamic8/1
  Selector9/1 -> Lookup Table Dynamic8/3
  Selector11/1 -> Lookup Table Dynamic11/3
  [Time] -> Lookup Table Dynamic11/1
  [TimeVec] -> Lookup Table Dynamic11/2
  [TimeVec] -> Lookup Table Dynamic10/2
  [Time] -> Lookup Table Dynamic10/1
  Selector12/1 -> Lookup Table Dynamic10/3
  Lookup Table Dynamic11/1 -> Mux1/12
  Lookup Table Dynamic10/1 -> Mux1/11
  Lookup Table Dynamic9/1 -> Mux1/10
  Lookup Table Dynamic8/1 -> Mux1/9
  Lookup Table Dynamic7/1 -> Mux1/8
  Lookup Table Dynamic6/1 -> Mux1/7

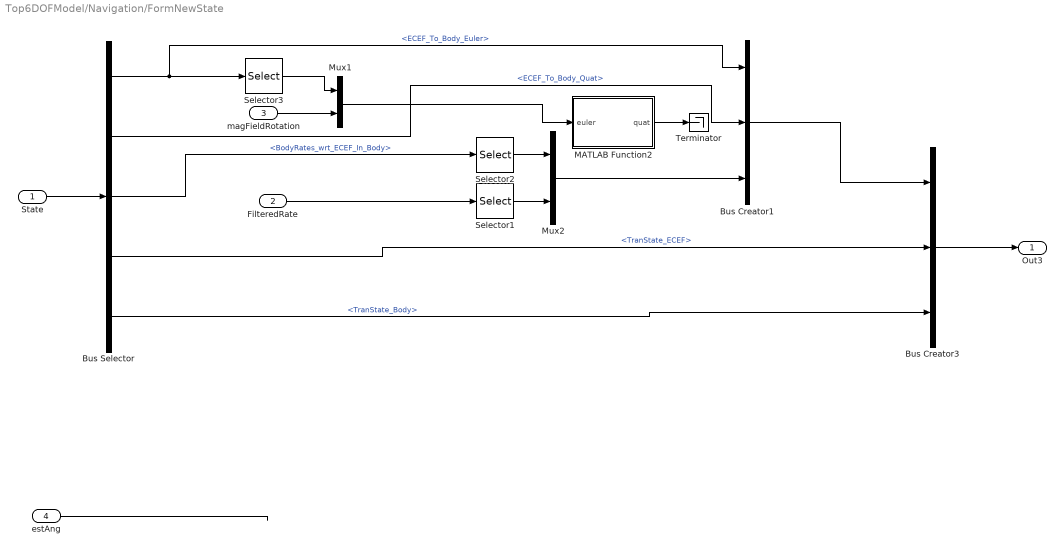
== system Top6DOFModel/Navigation/FormNewState ==
  State : Inport
  FilteredRate : Inport  Port=2
  magFieldRotation : Inport  Port=3
  estAng : Inport  Port=4
  Bus Creator1 : BusCreator  Inputs=3  OutDataTypeStr=Bus: RotStateBodyECEFBus
      settings: InheritFromInputs=off
  Bus Creator3 : BusCreator  Inputs=3  OutDataTypeStr=Bus: FullStateBus
      settings: InheritFromInputs=off
  Bus Selector : BusSelector  OutputSignals=RotState_Body_ECEF.ECEF_To_Body_Euler,RotState_Body_ECEF.ECEF_To_Body_Quat,RotState_Body_ECEF.BodyRates_wrt_ECEF_In_Body,TranState_ECEF,TranState_Body
  MATLAB Function2 : MATLAB Function  TreatAsAtomicUnit=on
  Mux1 : Mux  Inputs=2
  Mux2 : Mux  Inputs=2
  Selector1 : Selector  InputPortWidth=3  IndexOptions=Index vector (dialog)  Indices=3  OutputSizes=1
  Selector2 : Selector  InputPortWidth=3  IndexOptions=Index vector (dialog)  Indices=[1:2]  OutputSizes=1
  Selector3 : Selector  InputPortWidth=3  IndexOptions=Index vector (dialog)  Indices=[1:2]  OutputSizes=1
  Terminator : Terminator
  Out3 : Outport
  wires:
  State/1 -> Bus Selector/1
  Selector2/1 -> Mux2/1
  Bus Selector/3 -> Selector2/1  "<BodyRates_wrt_ECEF_In_Body>"
  Selector1/1 -> Mux2/2
  Bus Selector/5 -> Bus Creator3/3  "<TranState_Body>"
  FilteredRate/1 -> Selector1/1
  Bus Selector/4 -> Bus Creator3/2  "<TranState_ECEF>"
  Bus Creator3/1 -> Out3/1
  Mux2/1 -> Bus Creator1/3
  Bus Selector/1 -> Bus Creator1/1, Selector3/1  "<ECEF_To_Body_Euler>"
  Selector3/1 -> Mux1/1
  magFieldRotation/1 -> Mux1/2
  Mux1/1 -> MATLAB Function2/1(euler)
  Bus Creator1/1 -> Bus Creator3/1
  Bus Selector/2 -> Bus Creator1/2  "<ECEF_To_Body_Quat>"
  MATLAB Function2/1(quat) -> Terminator/1
  estAng/1 -> ?

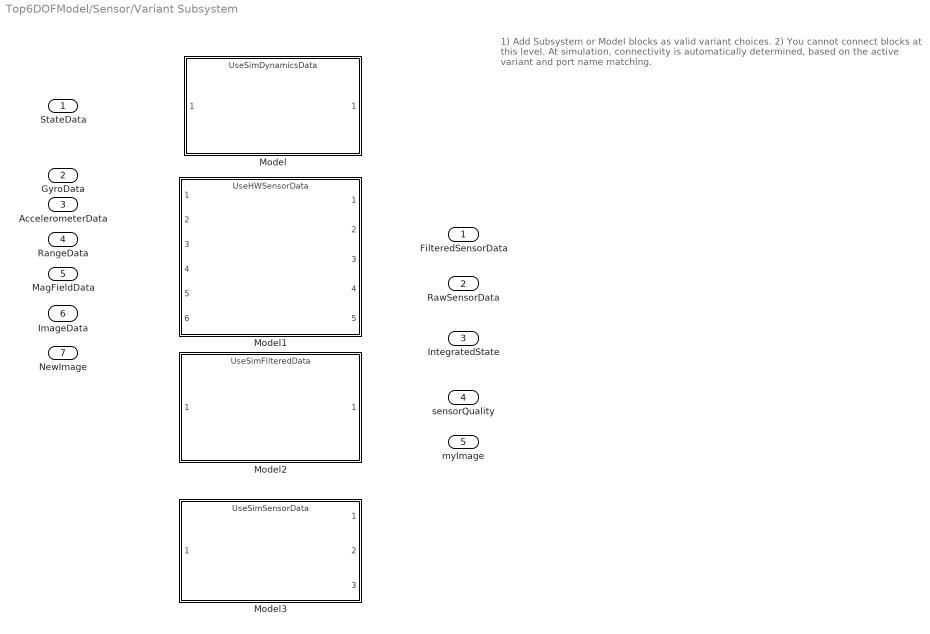
== system Top6DOFModel/Sensor/Variant Subsystem ==
  note: 1) Add Subsystem or Model blocks as valid variant choices.
      | 2) You cannot connect blocks at this level. At simulation, connectivity is automatically
      | determined, based on the active variant and port name matching.
  StateData : Inport
  GyroData : Inport  Port=2
  AccelerometerData : Inport  Port=3
  RangeData : Inport  Port=4  OutDataTypeStr=uint8
  MagFieldData : Inport  Port=5
  ImageData : Inport  Port=6
  NewImage : Inport  Port=7
  Model : ModelReference  ModelNameDialog=UseSimDynamicsData  SimulationMode=Normal  VariantControl=VSS_SIMDYNAMICS  ModelReferenceVersion=1.25
  Model1 : ModelReference  ModelNameDialog=UseHWSensorData  SimulationMode=Normal  VariantControl=VSS_HWSENSOR  ModelReferenceVersion=1.111
  Model2 : ModelReference  ModelNameDialog=UseSimFilteredData  SimulationMode=Normal  VariantControl=VSS_SIMFILTERED  ModelReferenceVersion=1.9
  Model3 : ModelReference  ModelNameDialog=UseSimSensorData  SimulationMode=Normal  VariantControl=VSS_SIMSENSOR  ModelReferenceVersion=1.51
  FilteredSensorData : Outport
  RawSensorData : Outport  Port=2
  IntegratedState : Outport  Port=3
  sensorQuality : Outport  Port=4
  myImage : Outport  Port=5  OutDataTypeStr=uint8

== matlab function Top6DOFModel/MATLAB Function ==
  data: m output; Izz output
function [m,Izz] = callplanarMassProperties

[m, Izz] = planarMassProperties();

== matlab function Top6DOFModel/IC_State/Form_ECEF_To_Body ==
  data: euler input; q output
function q  = fcn(euler)

q = EulerToquat_321(euler);

== matlab function Top6DOFModel/Compute_Outputs/Convert_Body_To_ECEF1/Form_ECEF_To_Body ==
  data: euler input; m output; q output
function [m,q] = fcn(euler)

m = EulerToDCM_321(euler);
q = EulerToquat_321(euler);

== matlab function Top6DOFModel/IC_State/Form_Body_Vec ==
  data: posECEF input; velECEF input; posBody output; velBody output; qin input
function [posBody,velBody] = fcn(posECEF,velECEF,qin)

posBody = quatrotate(posECEF,qin);
velBody = quatrotate(velECEF,qin);

== matlab function Top6DOFModel/Compute_Outputs/computeRangeData/MATLAB Function1 ==
  data: t input; range output; state input; rangeSensorLocBody input; rangeSensorAngBody input; rangeSensorFOV input; wallBounds input; rangeArray output
function [range,rangeArray] = callsenseWalls(t,state,rangeSensorLocBody,rangeSensorAngBody,rangeSensorFOV,wallBounds)

[range,rangeArray] = senseWalls(state,rangeSensorLocBody,rangeSensorAngBody,rangeSensorFOV,wallBounds);

== matlab function Top6DOFModel/Executive/MATLAB Function ==
  data: outControlMode output; navState input; refTraj input; inControlMode input
function outControlMode  = callgncExecutive(navState,refTraj,inControlMode)

[outControlMode] = gncExecutive(navState,refTraj,inControlMode);

== matlab function Top6DOFModel/Navigation/MATLAB Function ==
  data: rangeData input; estPos output
function estPos  = callestimatePosition(rangeData)

[estPos] = estimatePosition(rangeData);

== matlab function Top6DOFModel/MATLAB Function1 ==
  data: refTraj output; IC_State input
function refTraj   = callreferenceTrajectory(IC_State)

[refTraj] = referenceTrajectory(IC_State);

== matlab function Top6DOFModel/Navigation/FormNewState/MATLAB Function2 ==
  data: quat output; euler input
function quat  = computeQuat(euler)

quat = EulerToquat_321(euler);

== matlab function Top6DOFModel/Navigation/MATLAB Function1 ==
  data: thetaAng input; estAng output; targetVec input; cameraVec input
function estAng  = callestimateAttitude(thetaAng,targetVec,cameraVec)

[estAng] = estimateAttitude(thetaAng,targetVec,cameraVec);

== matlab function Top6DOFModel/Compute_Outputs/Convert_Body_To_ECEF2/Form_ECEF_To_Body ==
  data: euler input; m output; q output
function [m,q] = fcn(euler)

m = EulerToDCM_321(euler);
q = EulerToquat_321(euler);
